simulink model "MIPI3"  (R2024b)
settings: Solver=VariableStepAuto  StartTime=0.0  StopTime=1000  RelTol=1e-3
settings Model: Creator=emanuel-gifuni  LastModifiedBy=emanuel-gifuni

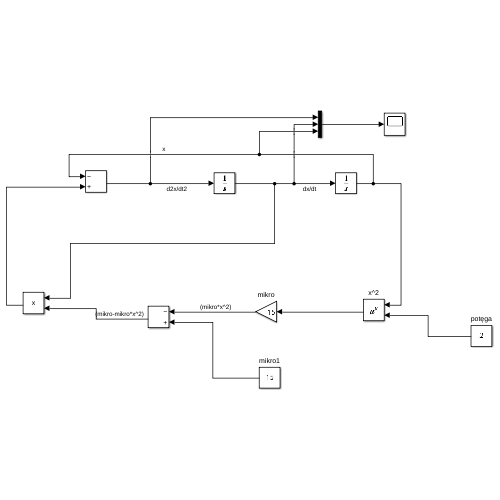
[thumbnail: Simulink's stored preview of the top-level diagram]
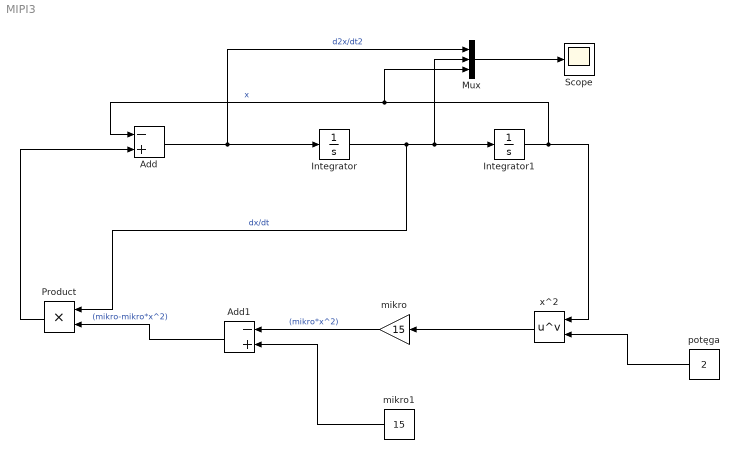
== system MIPI3 ==
  Add : Sum  Inputs=-+
  Add1 : Sum  Inputs=-+
  Integrator : Integrator  InitialCondition=1
  Integrator1 : Integrator  InitialCondition=2
  Mux : Mux  Inputs=3
  Product : Product
  Scope : Scope
  mikro : Gain  Gain=15
  mikro1 : Constant  Value=15
  potęga : Constant  Value=2
  x^2 : Math  Operator=pow
  wires:
  Add/1 -> Mux/1, Integrator/1  "d2x/dt2"
  Integrator/1 -> Product/1, Mux/2, Integrator1/1  "dx/dt"
  Integrator1/1 -> x^2/1, Mux/3, Add/1  "x"
  potęga/1 -> x^2/2
  x^2/1 -> mikro/1
  mikro/1 -> Add1/1  "(mikro*x^2)"
  mikro1/1 -> Add1/2
  Add1/1 -> Product/2  "(mikro-mikro*x^2)"
  Product/1 -> Add/2
  Mux/1 -> Scope/1
